simulink model "Gleichstrommotor_V1"  (Simulink 8.7)
settings: Solver=ode1  StartTime=0.0  StopTime=10  FixedStep=0.0001  RelTol=1e-3
values from neighbouring files (symbols this model uses):
  J_mot = 0.0001    [Gleichstrommotor_V1.m]
  k_mot = 0.03    [Gleichstrommotor_V1.m]
  L = 0.013    [Gleichstrommotor_V1.m]
  M_Last = 0.05    [Gleichstrommotor_V1.m]
  M_Reib = 0.01    [Gleichstrommotor_V1.m]
  R = 2    [Gleichstrommotor_V1.m]
  U = 12    [Gleichstrommotor_V1.m]
settings Model: Creator=Michaél  LastModifiedBy=Michaél
settings DataIOCC: LimitDataPoints=off  SaveFormat=Dataset
settings DebuggingCC: UnderspecifiedInitializationDetection=Simplified  MergeDetectMultiDrivingBlocksExec=error
settings HardwareCC: ProdBitPerPointer=64  ProdLargestAtomicFloat=Float  ProdIntDivRoundTo=Zero  ProdEndianess=LittleEndian  ProdWordSize=64  ProdHWDeviceType=Intel->x86-64 (Windows64)
settings ModelReferenceCC: PropagateSignalLabelsOutOfModel=on
settings ConfigComp: CovModelRefEnable=off

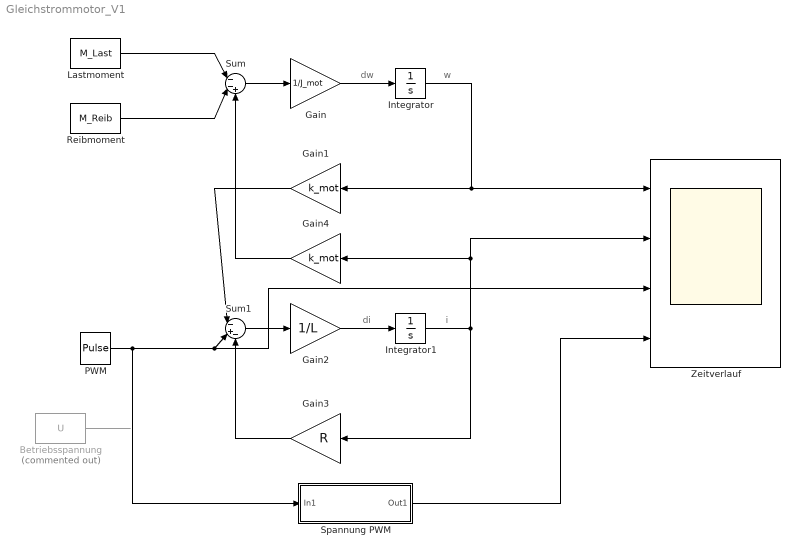
== system Gleichstrommotor_V1 ==
  note: w
  note: dw
  note: di
  note: i
  "Betriebsspannung " : Constant  Commented=on  Value=U
  Gain : Gain  Gain=1/J_mot
  Gain1 : Gain  Gain=k_mot
  Gain2 : Gain  Gain=1/L
  Gain3 : Gain  Gain=R
  Gain4 : Gain  Gain=k_mot
  Integrator : Integrator  LimitOutput=on  LowerSaturationLimit=0
  Integrator1 : Integrator
  Lastmoment : Constant  Value=M_Last
  PWM : DiscretePulseGenerator  PulseType=Time based  Amplitude=12  Period=0.001  PulseWidth=50
  Reibmoment : Constant  Value=M_Reib
  Spannung PWM : Subsystem
  Sum : Sum  Inputs=|--+
  Sum1 : Sum  Inputs=|-+-
  Zeitverlauf : Scope  NumInputPorts=4
  wires:
  Lastmoment/1 -> Sum/1
  Reibmoment/1 -> Sum/2
  Sum/1 -> Gain/1
  Gain/1 -> Integrator/1
  Integrator/1 -> Gain1/1, Zeitverlauf/1
  Gain1/1 -> Sum1/1
  Sum1/1 -> Gain2/1
  Gain2/1 -> Integrator1/1
  Integrator1/1 -> Gain4/1, Zeitverlauf/2, Gain3/1
  Gain3/1 -> Sum1/3
  Gain4/1 -> Sum/3
  PWM/1 -> Spannung PWM/1(In1), Zeitverlauf/3, Sum1/2
  Spannung PWM/1(Out1) -> Zeitverlauf/4
  "Betriebsspannung "/1 -> ?

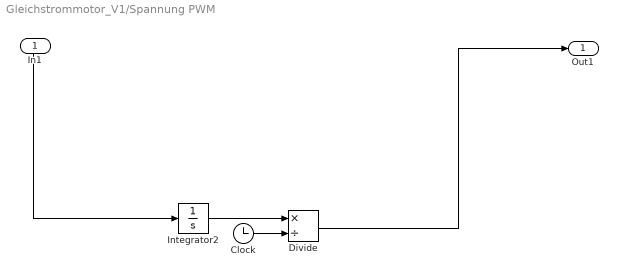
== system Gleichstrommotor_V1/Spannung PWM ==
  In1 : Inport
  Clock : Clock
  Divide : Product  Inputs=*/
  Integrator2 : Integrator
  Out1 : Outport
  wires:
  In1/1 -> Integrator2/1
  Integrator2/1 -> Divide/1
  Clock/1 -> Divide/2
  Divide/1 -> Out1/1
